simulink model "eVTOL_HIL"  (R2024b)
settings: Solver=FixedStepAuto  StartTime=0.0  StopTime=inf  FixedStep=SAMPLE_TIME  RelTol=1e-3
values from neighbouring files (symbols this model uses):
  aDl =     [initdata.mat]
  aDr =     [initdata.mat]
  aDyn =     [initdata.mat]
  aLat =     [initdata.mat]
  aLon =     [initdata.mat]
  D = Prop.D    [EOM_dt_MC.m]    (also in EOM_get_alf_dt_de_prop_evtol.m = CD * QS)
  General = init_layoutdata    [EOM_dt_MC.m]    (also in build_optimized_CA.m; initdata.mat = ; initdata_HIL_eVTOL.m)
  mass = Con(3)    [EOM_get_alf_dt_de_prop_evtol.m]    (also in initdata.mat = 2255.54; initdata_HIL_eVTOL.m = 7)
  Motor = init_motor_evtol    [EOM_dt_MC.m]    (also in initdata.mat = []; initdata_HIL_eVTOL.m)
  Prop = init_propeller_evtol_new    [EOM_dt_MC.m]    (also in initdata_HIL_eVTOL.m)
  SAMPLE_TIME = 0.01    [initdata_HIL_eVTOL.m]
undefined symbols (not defined in the file or in its folder): aDa, aDe, asbhl20env, Environment, InitData, magnitude
libraries: simulink_extras x16, vrlib x8, matrix_library x6, sharedutil x6, aerolibwindfilters x4, sharedtransform x4, aerolibfltsims x3, instrumentseriallib x3, uavmavlinklib x3, aerolibasang x3, aerolibobsolete x2, aerolibanimutils x1
(part 3 of 4)

== system eVTOL_HIL/eVTOL Dynamic Model/Energy & Power/thrust_6/Propeller  ==
  rpm : Inport
  V : Inport  Port=2
  rho : Inport  Port=3
  theta_b : Inport  Port=4
  D^5 : Constant  Value=5
  Diameter : Constant  Value=Prop.D
  Divide : Product  Inputs=4
  Divide2 : Product  Inputs=4
  Divide3 : Product  Inputs=**/
  Gain : Gain  Gain=1/60
  Math Function : Math  Operator=magnitude^2  SignedPower=on
  Math Function1 : Math  Operator=magnitude^2  SignedPower=on
  Math Function2 : Math  Operator=magnitude^2  SignedPower=on
  Math Function3 : Math  Operator=pow  SignedPower=on
  Math Function4 : Math  Operator=pow  SignedPower=on
  Scope{,1..4} (5 alike) : Scope
  Subsystem : Subsystem
  get CP : Lookup_n-D  BreakpointsForDimension1=Prop.J  BreakpointsForDimension2=Prop.theta_b  IndexSearchMethod=Linear search  BeginIndexSearchUsingPreviousIndexResult=on  Table=Prop.CP  RndMeth=Simplest
      settings: InputPortMap=u0,u1
  get CT : Lookup_n-D  BreakpointsForDimension1=Prop.J  BreakpointsForDimension2=Prop.theta_b  IndexSearchMethod=Linear search  BeginIndexSearchUsingPreviousIndexResult=on  Table=Prop.CT  RndMeth=Simplest
      settings: InputPortMap=u0,u1
  "n^3 " : Constant  Value=3
  P_plr (w) : Outport  VectorParamsAs1DForOutWhenUnconnected=off
  T (N) : Outport  Port=2  VectorParamsAs1DForOutWhenUnconnected=off
  eta_p : Outport  Port=3  VectorParamsAs1DForOutWhenUnconnected=off
  wires:
  Divide2/1 -> P_plr (w)/1, Scope/1
  Divide3/1 -> eta_p/1  "eta_p"
  D^5/1 -> Math Function4/2
  Math Function4/1 -> Divide2/4
  "n^3 "/1 -> Math Function3/2
  Math Function3/1 -> Divide2/3
  get CP/1 -> Divide3/3, Divide2/1, Scope3/1
  rpm/1 -> Gain/1, Subsystem/2(rpm)
  Subsystem/1(J) -> Scope2/1, get CT/1, Divide3/1, get CP/1
  Divide/1 -> Scope1/1, T (N)/1
  Math Function2/1 -> Divide/4  "D^4"
  Math Function1/1 -> Math Function2/1
  Diameter/1 -> Math Function1/1, Math Function4/1
  Math Function/1 -> Divide/3  "n^2"
  Gain/1 -> Math Function3/1, Math Function/1
  rho/1 -> Divide/2, Divide2/2
  get CT/1 -> Divide3/2, Divide/1, Scope4/1
  V/1 -> Subsystem/1(V)
  theta_b/1 -> get CP/2, get CT/2

== system eVTOL_HIL/eVTOL Dynamic Model/Environment/Wind Models/Dryden Wind Turbulence Model (Continuous (+q -r)) ==
  Altitude : Inport  Unit=m
  Airspeed : Inport  Port=2  Unit=m/s
  DCM : Inport  Port=3  Unit=1  PortDimensions=[3 3]
  (u,v,w) : Selector  InputPortWidth=4  IndexOptions=Index vector (dialog)  Indices=[1 2 3]  OutputSizes=1
  Angle Conversion : Subsystem
  Bus Creator : BusCreator  Inputs=3
  Cast : DataTypeConversion  SaturateOnIntegerOverflow=off  RndMeth=Floor
  Cast To Double{,1..4} (5 alike) : DataTypeConversion  OutDataTypeStr=double  SaturateOnIntegerOverflow=off  RndMeth=Floor
  Disallow CGS : UnitConfiguration  UnitSystemsStr=English,SI,SI (extended)  AllowAllUnitSystems=off
  Filters on angular rates : Subsystem  mask(Angular Rates){}
  Filters on velocities : aerolibwindfilters/Dryden Continuous Filters  SystemSampleTime=-1  VariantActivationTime=update diagram  AllowFlexibleInterface=on  Latency=0  AutoFrameSizeCalculation=off
  Length Conversion : Subsystem
  Length Conversion1 : Subsystem
  Mux : Mux  Inputs=3
  Mux1 : Mux  Inputs=3
  RMS turbulence intensities : Subsystem
  Select angular rates : Subsystem
  Select velocities : Subsystem
  Turbulence scale lengths : Subsystem
  Unit Conversion : UnitConversion  OutputType=Inherit: Inherit via back propagation
  Velocity Conversion : Subsystem
  Velocity Conversion2 : Subsystem
  White Noise : aerolibcommonsys/Tunable White Noise  pwr=[1 1 1 1]*pi  Ts=ts  seed=Seed
  Wind direction : Constant  Value=Wdeg
  Windspeed at 20ft (6m) : Constant  Value=W20
  Wingspan : Constant  Value=Wingspan
  p : Selector  InputPortWidth=4  IndexOptions=Index vector (dialog)  Indices=[4]  OutputSizes=1
  ug,vg,wg : Outport  Unit=m/s  VectorParamsAs1DForOutWhenUnconnected=off
  pg,qg,rg : Outport  Port=2  VectorParamsAs1DForOutWhenUnconnected=off
  wires:
  Cast To Double4/1 -> Velocity Conversion/1(in)
  Airspeed/1 -> Cast To Double4/1
  Cast To Double3/1 -> Length Conversion1/1(in)
  Wingspan/1 -> Cast To Double3/1
  Cast To Double2/1 -> Length Conversion/1(in)
  Cast To Double1/1 -> Angle Conversion/1(in)
  Cast To Double/1 -> Bus Creator/1  "DCM"
  Mux1/1 -> Cast/1
  Cast/1 -> pg,qg,rg/1
  (u,v,w)/1 -> Filters on velocities/1
  Unit Conversion/1 -> ug,vg,wg/1
  Velocity Conversion/1(out) -> Filters on angular rates/3(V), Filters on velocities/8
  Angle Conversion/1(out) -> Bus Creator/2  "Wdeg"
  Length Conversion1/1(out) -> Filters on angular rates/7(wingspan)
  Bus Creator/1 -> Select angular rates/4("DCM, altitude, Wdeg"), Select velocities/1("DCM, altitude, Wdeg")
  DCM/1 -> Cast To Double/1  "DCM"
  Wind direction/1 -> Cast To Double1/1
  Select angular rates/3(rgw) -> Mux1/3
  Select angular rates/2(qgw) -> Mux1/2
  Select angular rates/1(pgw) -> Mux1/1
  Select velocities/3(wgw) -> Mux/3
  Select velocities/2(vgw) -> Mux/2
  Select velocities/1(ugw) -> Mux/1
  Velocity Conversion2/1(out) -> RMS turbulence intensities/2(Windspeed at 20ft (6m))
  Windspeed at 20ft (6m)/1 -> Velocity Conversion2/1(in)
  RMS turbulence intensities/2(sigma_vg) -> Filters on velocities/6
  Filters on velocities/3 -> Filters on angular rates/2(wg), Select velocities/4(wgw_h&l)  "wgw"
  Filters on velocities/2 -> Filters on angular rates/1(vg), Select velocities/3(vgw_h&l)  "vgw"
  RMS turbulence intensities/1("sigma_ug ") -> Filters on velocities/5
  Filters on velocities/1 -> Select velocities/2(ugw_h&l)  "ugw"
  Filters on angular rates/3(rgw) -> Select angular rates/3(rgw_h&l)  "rgw"
  Filters on angular rates/2(qgw) -> Select angular rates/2(qgw_h&l)  "qgw"
  Filters on angular rates/1(pgw) -> Select angular rates/1(pgw_h&l)  "pgw"
  RMS turbulence intensities/3(sigma_wg) -> Filters on angular rates/5(sigma_w), Filters on velocities/7
  Turbulence scale lengths/3(L_wg) -> Filters on angular rates/4(Lw), Filters on velocities/4
  Turbulence scale lengths/1(L_ug) -> Filters on velocities/2
  Altitude/1 -> Cast To Double2/1
  Mux/1 -> Unit Conversion/1
  White Noise/1 -> (u,v,w)/1, p/1
  p/1 -> Filters on angular rates/6(Noise)
  Length Conversion/1(out) -> Bus Creator/3, RMS turbulence intensities/1(Altitude), Turbulence scale lengths/1(Altitude)  "altitude"
  Turbulence scale lengths/2(L_vg) -> Filters on velocities/3

== system eVTOL_HIL/eVTOL Dynamic Model/airframe/Flight Conditions/Subsystem2 ==
  Ve : Inport
  Dot Product1 : DotProduct  OutDataTypeStr=Inherit: Inherit via internal rule
  Gain1 : Gain  Gain=-1
  Selector4 : Selector  InputPortWidth=3  IndexOptions=Index vector (dialog)  Indices=3  OutputSizes=1
  Selector5 : Selector  InputPortWidth=3  IndexOptions=Index vector (dialog)  Indices=[1 2]  OutputSizes=1
  Selector6 : Selector  InputPortWidth=3  IndexOptions=Index vector (dialog)  Indices=2  OutputSizes=1
  Selector7 : Selector  InputPortWidth=3  IndexOptions=Index vector (dialog)  Indices=3  OutputSizes=1
  Sqrt1 : Sqrt
  Trigonometric Function2 : Trigonometry  Operator=atan2
  Trigonometric Function3 : Trigonometry  Operator=atan2
  gamma : Outport
  chi : Outport  Port=2
  wires:
  Ve/1 -> Selector7/1, Selector6/1, Selector5/1, Selector4/1
  Selector6/1 -> Trigonometric Function3/1
  Selector5/1 -> Dot Product1/1, Dot Product1/2
  Selector7/1 -> Trigonometric Function3/2
  Trigonometric Function2/1 -> gamma/1
  Gain1/1 -> Trigonometric Function2/1
  Dot Product1/1 -> Sqrt1/1
  Sqrt1/1 -> Trigonometric Function2/2
  Trigonometric Function3/1 -> chi/1
  Selector4/1 -> Gain1/1

== system eVTOL_HIL/eVTOL Dynamic Model/airframe/Flight Conditions/Vel in Inertial Axes ==
  Ve : Inport
  Demux : Demux  Outputs=3
  Dot Product1 : DotProduct  OutDataTypeStr=Inherit: Inherit via internal rule
  Fcn : Fcn  Expr=sqrt(u(1)^2+u(2)^2)
  Gain : Gain  Gain=3.6
  Mux : Mux  Inputs=2
  Mux1 : Mux  Inputs=5
  Sqrt : Sqrt
  Ve_Inertial : Outport  VectorParamsAs1DForOutWhenUnconnected=off
  wires:
  Demux/3 -> Mux1/3  "v_d"
  Ve/1 -> Demux/1, Dot Product1/2, Dot Product1/1
  Fcn/1 -> Mux1/4  "v_horizontal"
  Demux/1 -> Mux/1, Mux1/1  "v_n"
  Demux/2 -> Mux/2, Mux1/2  "v_e"
  Mux/1 -> Fcn/1
  Mux1/1 -> Ve_Inertial/1
  Gain/1 -> Mux1/5  "groundspeed(km/h)"
  Sqrt/1 -> Gain/1
  Dot Product1/1 -> Sqrt/1

== system eVTOL_HIL/eVTOL Dynamic Model/airframe/force moment/Gear&FM in body axis ==
  PlantData : Inport
  Add1 : Sum  Inputs=++++
  Add2 : Sum  Inputs=++++
  Constant1 : Constant  Value=0
  Constant6 : Constant  Value=0
  F 4 gear : Scope  NumInputPorts=4
  F&M  Front Gear Left : Subsystem
  F&M  Front Gear Right : Subsystem
  F&M  Main Gear Left : Subsystem
  F&M  Main Gear Right : Subsystem
  M 4 gear : Scope  NumInputPorts=4
  F_Gear : Outport  VectorParamsAs1DForOutWhenUnconnected=off
  M_Gear : Outport  Port=2  VectorParamsAs1DForOutWhenUnconnected=off
  wires:
  PlantData/1 -> F&M  Main Gear Right/1(PlantData), F&M  Main Gear Left/1(PlantData), F&M  Front Gear Right/1(PlantData), F&M  Front Gear Left/1(PlantData)
  F&M  Front Gear Left/2(M_fgl) -> M 4 gear/1, Add2/1
  F&M  Front Gear Left/1(F_fgl) -> F 4 gear/1, Add1/1
  F&M  Front Gear Right/1(F_fgl) -> F 4 gear/2, Add1/2
  F&M  Main Gear Left/1(F_fgl) -> F 4 gear/3, Add1/3
  F&M  Main Gear Right/1(F_fgl) -> F 4 gear/4, Add1/4
  Add1/1 -> F_Gear/1
  F&M  Front Gear Right/2(M_fgl) -> M 4 gear/2, Add2/2
  F&M  Main Gear Left/2(M_fgl) -> M 4 gear/3, Add2/3
  F&M  Main Gear Right/2(M_fgl) -> M 4 gear/4, Add2/4
  Add2/1 -> M_Gear/1
  Constant6/1 -> F&M  Main Gear Left/2(dg)
  Constant1/1 -> F&M  Main Gear Right/2(dg)

== system eVTOL_HIL/eVTOL Dynamic Model/airframe/force moment/Thrust&M in body axis ==
  prop : Inport
  3x3 Cross Product{,1..5} (6 alike) : sharedutil/3x3 Cross Product  aMode=aMode
  Bus Selector1 : BusSelector  OutputSignals=T_1,T_2,T_3,T_4,T_5,T_6,Q
  Constant1 : Constant  Value=General.pos_plr3
  Constant2 : Constant  Value=General.pos_plr4
  Constant3 : Constant  Value=General.pos_plr5
  Constant4 : Constant  Value=General.pos_plr1
  Constant5 : Constant  Value=General.pos_plr6
  Constant6 : Constant  Value=General.pos_plr2
  Display3 : Display
  Scope2 : Scope
  Sum2 : Sum  Inputs=++++++
  Sum3 : Sum  Inputs=++++++
  Sum4 : Sum  Inputs=++|
  T MC : Scope  NumInputPorts=6
  f_T : Outport  VectorParamsAs1DForOutWhenUnconnected=off
  m_T : Outport  Port=2  VectorParamsAs1DForOutWhenUnconnected=off
  wires:
  prop/1 -> Bus Selector1/1
  Constant4/1 -> 3x3 Cross Product/1
  Constant6/1 -> 3x3 Cross Product1/1
  Constant1/1 -> 3x3 Cross Product2/1
  Constant2/1 -> 3x3 Cross Product3/1
  Bus Selector1/1 -> T MC/1, [T_1]  "<T_1>"
  Bus Selector1/2 -> [T_2], T MC/2  "<T_2>"
  Bus Selector1/3 -> [T_3], T MC/3  "<T_3>"
  Bus Selector1/4 -> [T_4], T MC/4  "<T_4>"
  [T_1] -> 3x3 Cross Product/2
  [T_2] -> 3x3 Cross Product1/2
  [T_3] -> 3x3 Cross Product2/2
  [T_4] -> 3x3 Cross Product3/2
  [T_1] -> Sum2/1
  [T_2] -> Sum2/2
  [T_3] -> Sum2/3
  [T_4] -> Sum2/4
  3x3 Cross Product/1 -> Sum3/1
  3x3 Cross Product1/1 -> Sum3/2
  3x3 Cross Product2/1 -> Sum3/3
  3x3 Cross Product3/1 -> Sum3/4
  Sum2/1 -> f_T/1, Scope2/1, Display3/1  "T"
  Sum3/1 -> Sum4/2
  Bus Selector1/5 -> [T_5], T MC/5  "<T_5>"
  Sum4/1 -> m_T/1
  [Q] -> Sum4/1
  Bus Selector1/6 -> T MC/6, [T_6]  "<T_6>"
  Bus Selector1/7 -> [Q]  "<Q>"
  [T_5] -> Sum2/5
  [T_6] -> Sum2/6
  [T_5] -> 3x3 Cross Product4/2
  3x3 Cross Product4/1 -> Sum3/5
  Constant3/1 -> 3x3 Cross Product4/1
  [T_6] -> 3x3 Cross Product5/2
  3x3 Cross Product5/1 -> Sum3/6
  Constant5/1 -> 3x3 Cross Product5/1

== system eVTOL_HIL/eVTOL Dynamic Model/airframe/force moment/aero F&M in body axis ==
  PlantData : Inport
  Act_surface : Inport  Port=2
  Aerodynamic Coefficients : Subsystem  AncestorBlock=asbhl20vehicle/Vehicle/Aerodynamic/Aerodynamic Coefficients
      settings: LibrarySourceBlock=|
      | asbhl20vehicle/Vehicle/Aerodynamic/Aerodynamic
      | Coefficients
  "Aerodynamic Forces and Moments " : aerolibadyn/Aerodynamic Forces and Moments   inputAxes=Body  outputForceAxes=Body  outputMomentAxes=Body  S=General.Sw  b=General.b  cbar=General.MAC
  Center of Gravity : Constant  Value=[0 0 0]  SampleTime=0
  Center of Pressure : Constant  Value=[0 0 0]  SampleTime=0
  Constant : Constant
  Constant1 : Constant  Commented=on
  Mux1 : Mux  Inputs=2
  PlantBus : BusSelector  OutputSignals=Vb,alpha,beta,pqr,Va,alphaDot,mach
  PlantBus1 : BusSelector  OutputSignals=DynamicPressure
  PlantData_1 : InportShadow
  Product : Product
  Product1 : Product
  Scope1 : Scope  Commented=on
  Scope2 : Scope
  Scope3 : Scope
  Scope4 : Scope  Commented=on
  Selector : Selector  Commented=on  InputPortWidth=3  IndexOptions=Index vector (dialog)  Indices=1  OutputSizes=1
  Switch : Switch  Commented=on  Criteria=u2 > Threshold  Threshold=3  SaturateOnIntegerOverflow=off  InputSameDT=off
  nonunit value : Subsystem
  Fb (X Y Z) : Outport  VectorParamsAs1DForOutWhenUnconnected=off
  M (L M N) : Outport  Port=2  VectorParamsAs1DForOutWhenUnconnected=off
  wires:
  "Aerodynamic Forces and Moments "/1 -> Product/1, Scope2/1
  "Aerodynamic Forces and Moments "/2 -> Product1/1, Scope3/1
  PlantData/1 -> PlantBus/1
  Act_surface/1 -> Aerodynamic Coefficients/5(Act_surface)
  PlantBus/2 -> Mux1/1  "<alpha>"
  PlantBus/3 -> Mux1/2  "<beta>"
  PlantBus/4 -> nonunit value/2(pqr)  "<pqr>"
  Center of Gravity/1 -> "Aerodynamic Forces and Moments "/3
  Center of Pressure/1 -> "Aerodynamic Forces and Moments "/4
  PlantData_1/1 -> PlantBus1/1
  PlantBus/6 -> nonunit value/3(alphaDot)  "<alphaDot>"
  PlantBus/5 -> nonunit value/1(V)  "<Va>"
  Constant1/1 -> Switch/1
  Constant/1 -> [Aero_SW]
  Switch/1 -> Scope1/1
  Product/1 -> Fb (X Y Z)/1
  Product1/1 -> M (L M N)/1
  [Aero_SW] -> Product/2
  [Aero_SW] -> Product1/2
  PlantBus/1 -> Selector/1  "<Vb>"
  Selector/1 -> Switch/2, Scope4/1  "Vb_x"
  Mux1/1 -> Aerodynamic Coefficients/1(Incid)
  nonunit value/1(pqr_n) -> Aerodynamic Coefficients/3(pqrn)
  nonunit value/2(alphaDot_n) -> Aerodynamic Coefficients/4(alphaDot_n)
  Aerodynamic Coefficients/1(Coeff) -> "Aerodynamic Forces and Moments "/1
  PlantBus/7 -> Aerodynamic Coefficients/2(mach)  "<mach>"
  PlantBus1/1 -> "Aerodynamic Forces and Moments "/2  "<DynamicPressure>"

== system eVTOL_HIL/eVTOL Dynamic Model/airframe/force moment/gravity in body axis ==
  PlantData : Inport
  EnvmData : Inport  Port=2
  Bus Selector1 : BusSelector  OutputSignals=DCM_be,mass
  Bus Selector2 : BusSelector  OutputSignals=g
  G in body axis : Product  Multiplication=Matrix(*)  RndMeth=Zero
  Gain1 : Gain  Gain=[0; 0; 1]
  Product : Product  RndMeth=Zero
  Fb : Outport  VectorParamsAs1DForOutWhenUnconnected=off
  wires:
  Bus Selector1/1 -> G in body axis/1  "<DCM_be>"
  Gain1/1 -> G in body axis/2
  Bus Selector1/2 -> Product/1  "<mass>"
  Bus Selector2/1 -> Product/2  "<g>"
  Product/1 -> Gain1/1  "mg"
  PlantData/1 -> Bus Selector1/1
  G in body axis/1 -> Fb/1
  EnvmData/1 -> Bus Selector2/1

== system eVTOL_HIL/eVTOL Dynamic Model/Energy & Power/thrust_1/Propeller /Subsystem ==
  V : Inport
  rpm : Inport  Port=2
  Diameter : Constant  Value=Prop.D
  Divide : Product  Inputs=*//
  Gain : Gain  Gain=1/60
  J : Outport  VectorParamsAs1DForOutWhenUnconnected=off
  wires:
  Divide/1 -> J/1
  V/1 -> Divide/1
  rpm/1 -> Gain/1
  Gain/1 -> Divide/3  "rps"
  Diameter/1 -> Divide/2

== system eVTOL_HIL/eVTOL Dynamic Model/Energy & Power/thrust_2/Propeller /Subsystem ==
  V : Inport
  rpm : Inport  Port=2
  Diameter : Constant  Value=Prop.D
  Divide : Product  Inputs=*//
  Gain : Gain  Gain=1/60
  J : Outport  VectorParamsAs1DForOutWhenUnconnected=off
  wires:
  Divide/1 -> J/1
  V/1 -> Divide/1
  rpm/1 -> Gain/1
  Gain/1 -> Divide/3  "rps"
  Diameter/1 -> Divide/2

== system eVTOL_HIL/eVTOL Dynamic Model/Energy & Power/thrust_3/Propeller /Subsystem ==
  V : Inport
  rpm : Inport  Port=2
  Diameter : Constant  Value=Prop.D
  Divide : Product  Inputs=*//
  Gain : Gain  Gain=1/60
  J : Outport  VectorParamsAs1DForOutWhenUnconnected=off
  wires:
  Divide/1 -> J/1
  V/1 -> Divide/1
  rpm/1 -> Gain/1
  Gain/1 -> Divide/3  "rps"
  Diameter/1 -> Divide/2

== system eVTOL_HIL/eVTOL Dynamic Model/Energy & Power/thrust_4/Propeller /Subsystem ==
  V : Inport
  rpm : Inport  Port=2
  Diameter : Constant  Value=Prop.D
  Divide : Product  Inputs=*//
  Gain : Gain  Gain=1/60
  J : Outport  VectorParamsAs1DForOutWhenUnconnected=off
  wires:
  Divide/1 -> J/1
  V/1 -> Divide/1
  rpm/1 -> Gain/1
  Gain/1 -> Divide/3  "rps"
  Diameter/1 -> Divide/2

== system eVTOL_HIL/eVTOL Dynamic Model/Energy & Power/thrust_5/Propeller /Subsystem ==
  V : Inport
  rpm : Inport  Port=2
  Diameter : Constant  Value=Prop.D
  Divide : Product  Inputs=*//
  Gain : Gain  Gain=1/60
  J : Outport  VectorParamsAs1DForOutWhenUnconnected=off
  wires:
  Divide/1 -> J/1
  V/1 -> Divide/1
  rpm/1 -> Gain/1
  Gain/1 -> Divide/3  "rps"
  Diameter/1 -> Divide/2

== system eVTOL_HIL/eVTOL Dynamic Model/Energy & Power/thrust_6/Propeller /Subsystem ==
  V : Inport
  rpm : Inport  Port=2
  Diameter : Constant  Value=Prop.D
  Divide : Product  Inputs=*//
  Gain : Gain  Gain=1/60
  J : Outport  VectorParamsAs1DForOutWhenUnconnected=off
  wires:
  Divide/1 -> J/1
  V/1 -> Divide/1
  rpm/1 -> Gain/1
  Gain/1 -> Divide/3  "rps"
  Diameter/1 -> Divide/2

== system eVTOL_HIL/eVTOL Dynamic Model/Environment/Wind Models/Dryden Wind Turbulence Model (Continuous (+q -r))/Angle Conversion ==
  in : Inport  Unit=deg
  Unit Conversion : UnitConversion
  out : Outport  Unit=rad  VectorParamsAs1DForOutWhenUnconnected=off
  wires:
  in/1 -> Unit Conversion/1
  Unit Conversion/1 -> out/1

== system eVTOL_HIL/eVTOL Dynamic Model/Environment/Wind Models/Dryden Wind Turbulence Model (Continuous (+q -r))/Filters on angular rates ==
  vg : Inport
  wg : Inport  Port=2
  V : Inport  Port=3  Unit=ft/s
  Lw : Inport  Port=4
  sigma_w : Inport  Port=5
  Noise : Inport  Port=6
  wingspan : Inport  Port=7
  Constant1 : Constant  Value=T_on
  Constant2 : Constant  Value=T_on
  Constant3 : Constant  Value=T_on
  Hpgw : aerolibwindfilters/Hpgw(s)  SystemSampleTime=-1  VariantActivationTime=update diagram  AllowFlexibleInterface=on  Latency=0  AutoFrameSizeCalculation=off
  Hqgw : aerolibwindfilters/Hqgw(s) (+q)  SystemSampleTime=-1  VariantActivationTime=update diagram  AllowFlexibleInterface=on  Latency=0  AutoFrameSizeCalculation=off
  Hrgw : aerolibwindfilters/Hrgw(s) (-r)  SystemSampleTime=-1  VariantActivationTime=update diagram  AllowFlexibleInterface=on  Latency=0  AutoFrameSizeCalculation=off
  pgw : Outport  InitialOutput=0  VectorParamsAs1DForOutWhenUnconnected=off
  qgw : Outport  Port=2  InitialOutput=0  VectorParamsAs1DForOutWhenUnconnected=off
  rgw : Outport  Port=3  InitialOutput=0  VectorParamsAs1DForOutWhenUnconnected=off
  wires:
  Constant3/1 -> Hrgw/Enable
  Constant2/1 -> Hqgw/Enable
  Constant1/1 -> Hpgw/Enable
  Noise/1 -> Hpgw/3
  Lw/1 -> Hpgw/1
  sigma_w/1 -> Hpgw/2
  V/1 -> Hpgw/4, Hqgw/1, Hrgw/1
  Hpgw/1 -> pgw/1
  wg/1 -> Hqgw/2
  Hqgw/1 -> qgw/1
  Hrgw/1 -> rgw/1
  vg/1 -> Hrgw/2
  wingspan/1 -> Hqgw/3, Hrgw/3, Hpgw/5

== system eVTOL_HIL/eVTOL Dynamic Model/Environment/Wind Models/Dryden Wind Turbulence Model (Continuous (+q -r))/Length Conversion ==
  in : Inport
  Unit Conversion : UnitConversion
  out : Outport  Unit=ft  VectorParamsAs1DForOutWhenUnconnected=off
  wires:
  in/1 -> Unit Conversion/1
  Unit Conversion/1 -> out/1

== system eVTOL_HIL/eVTOL Dynamic Model/Environment/Wind Models/Dryden Wind Turbulence Model (Continuous (+q -r))/Length Conversion1 ==
  in : Inport  Unit=m
  Unit Conversion : UnitConversion
  out : Outport  Unit=ft  VectorParamsAs1DForOutWhenUnconnected=off
  wires:
  in/1 -> Unit Conversion/1
  Unit Conversion/1 -> out/1

== system eVTOL_HIL/eVTOL Dynamic Model/Environment/Wind Models/Dryden Wind Turbulence Model (Continuous (+q -r))/RMS turbulence intensities ==
  Altitude : Inport
  Windspeed at 20ft (6m) : Inport  Port=2
  High Altitude Intensity : Subsystem
  Low Altitude Intensity : Subsystem
  Mux1 : Mux  Inputs=2
  Mux2 : Mux  Inputs=2
  "sigma_ug " : Outport  VectorParamsAs1DForOutWhenUnconnected=off
  sigma_vg : Outport  Port=2  VectorParamsAs1DForOutWhenUnconnected=off
  sigma_wg : Outport  Port=3  VectorParamsAs1DForOutWhenUnconnected=off
  wires:
  Mux2/1 -> sigma_vg/1, "sigma_ug "/1  "sigmaug"
  Windspeed at 20ft (6m)/1 -> Low Altitude Intensity/1(Windspeed at 20ft (6m))
  High Altitude Intensity/1(sigma_ug sigma_vg sigma_wg) -> Mux2/2, Mux1/2
  Mux1/1 -> sigma_wg/1  "sigmawg"
  Low Altitude Intensity/2(sigma_wg) -> Mux1/1
  Low Altitude Intensity/1(sigma_ug sigma_vg) -> Mux2/1
  Altitude/1 -> High Altitude Intensity/1(h), Low Altitude Intensity/2(h)

== system eVTOL_HIL/eVTOL Dynamic Model/Environment/Wind Models/Dryden Wind Turbulence Model (Continuous (+q -r))/Select angular rates ==
  pgw_h&l : Inport
  qgw_h&l : Inport  Port=2
  rgw_h&l : Inport  Port=3
  "DCM, altitude, Wdeg" : Inport  Port=4
  Bus Creator : BusCreator  Inputs=6
  Bus Selector : BusSelector  OutputSignals=pgw,qgw,rgw
  Bus Selector1 : BusSelector  OutputSignals=pgw,qgw,rgw,DCM,Wdeg,altitude
  Bus Selector2 : BusSelector  OutputSignals=DCM,pgw,qgw,rgw,Wdeg
  Bus Selector3 : BusSelector  OutputSignals=altitude,DCM,Wdeg
  Interpolate rates : Subsystem  TreatAsAtomicUnit=on
  Low altitude rates : Subsystem  TreatAsAtomicUnit=on
  Medium/High altitude rates : Subsystem  TreatAsAtomicUnit=on
  Merge Subsystems : Subsystem
  "if Height < Max low altitude elseif Height > Min isotropic altitude " : If  IfExpression=u1<=max_height_low  ElseIfExpressions=u1>=min_height_high
  pgw : Outport  InitialOutput=0  VectorParamsAs1DForOutWhenUnconnected=off
  qgw : Outport  Port=2  InitialOutput=0  VectorParamsAs1DForOutWhenUnconnected=off
  rgw : Outport  Port=3  InitialOutput=0  VectorParamsAs1DForOutWhenUnconnected=off
  wires:
  "DCM, altitude, Wdeg"/1 -> Bus Selector3/1
  Bus Selector3/1 -> Bus Creator/1, "if Height < Max low altitude elseif Height > Min isotropic altitude "/1  "<altitude>"
  Bus Creator/1 -> Bus Selector2/1, Bus Selector1/1, Bus Selector/1
  Bus Selector3/2 -> Bus Creator/2  "<DCM>"
  pgw_h&l/1 -> Bus Creator/3
  qgw_h&l/1 -> Bus Creator/4
  rgw_h&l/1 -> Bus Creator/5
  Bus Selector1/1 -> Interpolate rates/1(pgw_h&l)  "<pgw>"
  Bus Selector1/2 -> Interpolate rates/2(qgw_h&l)  "<qgw>"
  Bus Selector1/3 -> Interpolate rates/3(rgw_h&l)  "<rgw>"
  Bus Selector1/4 -> Interpolate rates/4(DCM)  "<DCM>"
  Bus Selector1/6 -> Interpolate rates/6(Altitude)  "<altitude>"
  Bus Selector2/1 -> Low altitude rates/1(DCM)  "<DCM>"
  Bus Selector2/2 -> Low altitude rates/2(pgw_h&l)  "<pgw>"
  Bus Selector2/3 -> Low altitude rates/3(qgw_h&l)  "<qgw>"
  Bus Selector2/4 -> Low altitude rates/4(rgw_h&l)  "<rgw>"
  Bus Selector/1 -> Medium/High altitude rates/1(pgw_h&l)  "<pgw>"
  Bus Selector/2 -> Medium/High altitude rates/2(qgw_h&l)  "<qgw>"
  Bus Selector/3 -> Medium/High altitude rates/3(rgw_h&l)  "<rgw>"
  Merge Subsystems/1(pgw) -> pgw/1
  Merge Subsystems/2(qgw) -> qgw/1
  Merge Subsystems/3(rgw) -> rgw/1
  Interpolate rates/1(pgw,qgw,rgw) -> Merge Subsystems/3(interpolated)
  Bus Selector3/3 -> Bus Creator/6  "<Wdeg>"
  Bus Selector2/5 -> Low altitude rates/5(Wind direction)  "<Wdeg>"
  Bus Selector1/5 -> Interpolate rates/5(Wind direction)  "<Wdeg>"
  "if Height < Max low altitude elseif Height > Min isotropic altitude "/1 -> [IF]
  [IF] -> Low altitude rates/Action
  "if Height < Max low altitude elseif Height > Min isotropic altitude "/2 -> [ELSEIF]
  [ELSEIF] -> Medium/High altitude rates/Action
  [ELSE] -> Interpolate rates/Action
  "if Height < Max low altitude elseif Height > Min isotropic altitude "/3 -> [ELSE]
  Medium/High altitude rates/1(pgw,qgw,rgw) -> Merge Subsystems/2(high)
  Low altitude rates/1(pgw,qgw,rgw) -> Merge Subsystems/1(low)

== system eVTOL_HIL/eVTOL Dynamic Model/Environment/Wind Models/Dryden Wind Turbulence Model (Continuous (+q -r))/Select velocities ==
  "DCM, altitude, Wdeg" : Inport
  ugw_h&l : Inport  Port=2
  vgw_h&l : Inport  Port=3
  wgw_h&l : Inport  Port=4
  Bus Creator : BusCreator  Inputs=6
  Bus Selector : BusSelector  OutputSignals=ugw,vgw,wgw
  Bus Selector1 : BusSelector  OutputSignals=ugw,vgw,wgw,DCM,Wdeg,altitude
  Bus Selector2 : BusSelector  OutputSignals=DCM,ugw,vgw,wgw,Wdeg
  Bus Selector3 : BusSelector  OutputSignals=altitude,DCM,Wdeg
  Interpolate velocities : Subsystem  TreatAsAtomicUnit=on
  Low altitude velocities : Subsystem  TreatAsAtomicUnit=on
  Medium/High altitude velocities : Subsystem  TreatAsAtomicUnit=on
  Merge Subsystems : Subsystem
  "if Height < Max low altitude elseif Height > Min isotropic altitude " : If  IfExpression=u1<=max_height_low  ElseIfExpressions=u1>=min_height_high
  ugw : Outport  Unit=ft/s  InitialOutput=0  VectorParamsAs1DForOutWhenUnconnected=off
  vgw : Outport  Port=2  Unit=ft/s  InitialOutput=0  VectorParamsAs1DForOutWhenUnconnected=off
  wgw : Outport  Port=3  Unit=ft/s  InitialOutput=0  VectorParamsAs1DForOutWhenUnconnected=off
  wires:
  "DCM, altitude, Wdeg"/1 -> Bus Selector3/1
  Bus Selector1/6 -> Interpolate velocities/6(Altitude)  "<altitude>"
  Low altitude velocities/1(ugw,vgw,wgw) -> Merge Subsystems/1(low)
  Medium/High altitude velocities/1(ugw,vgw,wgw) -> Merge Subsystems/2(high)
  "if Height < Max low altitude elseif Height > Min isotropic altitude "/3 -> [ELSE]
  [ELSE] -> Interpolate velocities/Action
  [ELSEIF] -> Medium/High altitude velocities/Action
  "if Height < Max low altitude elseif Height > Min isotropic altitude "/2 -> [ELSEIF]
  [IF] -> Low altitude velocities/Action
  "if Height < Max low altitude elseif Height > Min isotropic altitude "/1 -> [IF]
  Bus Selector1/5 -> Interpolate velocities/5(Wind direction)  "<Wdeg>"
  Bus Selector2/5 -> Low altitude velocities/5(Wind direction)  "<Wdeg>"
  Bus Selector3/3 -> Bus Creator/6  "<Wdeg>"
  Interpolate velocities/1(ugw,vgw,wgw) -> Merge Subsystems/3(interpolated)
  Merge Subsystems/3(wgw) -> wgw/1
  Merge Subsystems/2(vgw) -> vgw/1
  Merge Subsystems/1(ugw) -> ugw/1
  Bus Selector/3 -> Medium/High altitude velocities/3(wgw_h&l)  "<wgw>"
  Bus Selector/2 -> Medium/High altitude velocities/2(vgw_h&l)  "<vgw>"
  Bus Selector/1 -> Medium/High altitude velocities/1(ugw_h&l)  "<ugw>"
  Bus Selector2/4 -> Low altitude velocities/4(wgw_h&l)  "<wgw>"
  Bus Selector2/3 -> Low altitude velocities/3(vgw_h&l)  "<vgw>"
  Bus Selector2/2 -> Low altitude velocities/2(ugw_h&l)  "<ugw>"
  Bus Selector2/1 -> Low altitude velocities/1(DCM)  "<DCM>"
  Bus Selector1/4 -> Interpolate velocities/4(DCM)  "<DCM>"
  Bus Selector1/3 -> Interpolate velocities/3(wgw_h&l)  "<wgw>"
  Bus Selector1/2 -> Interpolate velocities/2(vgw_h&l)  "<vgw>"
  Bus Selector1/1 -> Interpolate velocities/1(ugw_h&l)  "<ugw>"
  wgw_h&l/1 -> Bus Creator/5
  vgw_h&l/1 -> Bus Creator/4
  ugw_h&l/1 -> Bus Creator/3
  Bus Selector3/2 -> Bus Creator/2  "<DCM>"
  Bus Creator/1 -> Bus Selector2/1, Bus Selector/1, Bus Selector1/1
  Bus Selector3/1 -> Bus Creator/1, "if Height < Max low altitude elseif Height > Min isotropic altitude "/1  "<altitude>"

== system eVTOL_HIL/eVTOL Dynamic Model/Environment/Wind Models/Dryden Wind Turbulence Model (Continuous (+q -r))/Turbulence scale lengths ==
  Altitude : Inport
  Low altitude scale length : Subsystem
  Lv : Gain  SaturateOnIntegerOverflow=on  OutDataTypeStr=Inherit: Same as input  ParamDataTypeStr=Inherit: Same as input
  Lw : Gain  SaturateOnIntegerOverflow=on  OutDataTypeStr=Inherit: Same as input  ParamDataTypeStr=Inherit: Same as input
  Medium/High altitude scale length : Subsystem
  Mux : Mux  Inputs=2
  Mux1 : Mux  Inputs=2
  L_ug : Outport  VectorParamsAs1DForOutWhenUnconnected=off
  L_vg : Outport  Port=2  VectorParamsAs1DForOutWhenUnconnected=off
  L_wg : Outport  Port=3  VectorParamsAs1DForOutWhenUnconnected=off
  wires:
  Lv/1 -> L_vg/1
  Lw/1 -> L_wg/1
  Altitude/1 -> Low altitude scale length/1(h)
  Mux/1 -> Lw/1  "Lwg"
  Mux1/1 -> Lv/1, L_ug/1  "Lug"
  Low altitude scale length/1(L_ug L_vg) -> Mux1/1
  Low altitude scale length/2(L_wg) -> Mux/1
  Medium/High altitude scale length/1(L_ug L_vg L_wg) -> Mux1/2, Mux/2

== system eVTOL_HIL/eVTOL Dynamic Model/Environment/Wind Models/Dryden Wind Turbulence Model (Continuous (+q -r))/Velocity Conversion ==
  in : Inport
  Unit Conversion : UnitConversion
  out : Outport  Unit=ft/s  VectorParamsAs1DForOutWhenUnconnected=off
  wires:
  in/1 -> Unit Conversion/1
  Unit Conversion/1 -> out/1

== system eVTOL_HIL/eVTOL Dynamic Model/Environment/Wind Models/Dryden Wind Turbulence Model (Continuous (+q -r))/Velocity Conversion2 ==
  in : Inport  Unit=m/s
  Unit Conversion : UnitConversion
  out : Outport  Unit=ft/s  VectorParamsAs1DForOutWhenUnconnected=off
  wires:
  in/1 -> Unit Conversion/1
  Unit Conversion/1 -> out/1

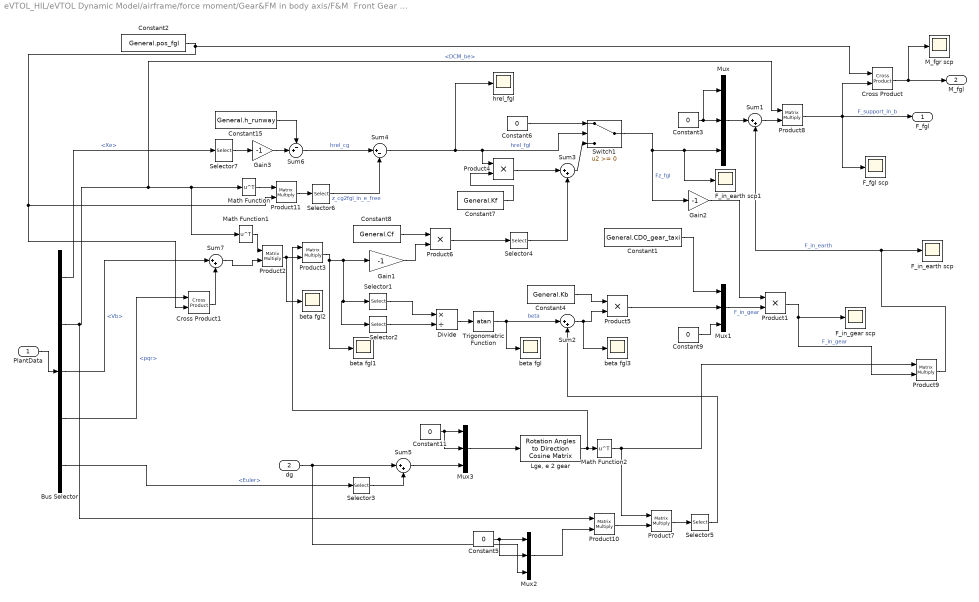
== system eVTOL_HIL/eVTOL Dynamic Model/airframe/force moment/Gear&FM in body axis/F&M  Front Gear Left ==
  PlantData : Inport
  dg : Inport  Port=2
  Bus Selector : BusSelector  OutputSignals=Xe,DCM_be,Vb,pqr,Euler
  Constant1 : Constant  Value=General.CD0_gear_taxi
  Constant{3,5..6,9,11} (5 alike) : Constant  Value=0
  Constant15 : Constant  Value=General.h_runway
  Constant2 : Constant  Value=General.pos_fgl
  Constant4 : Constant  Value=General.Kb
  Constant7 : Constant  Value=General.Kf
  Constant8 : Constant  Value=General.Cf
  Cross Product : vrlib/Utilities/Cross Product
  Cross Product1 : vrlib/Utilities/Cross Product
  Divide : Product  Inputs=*/
  F_fgl scp : Scope
  F_in_earth scp : Scope
  F_in_earth scp1 : Scope
  F_in_gear scp : Scope
  Gain1 : Gain  Gain=-1
  Gain2 : Gain  Gain=-1
  Gain3 : Gain  Gain=-1
  "Lge, e 2 gear" : sharedtransform/Rotation Angles to Direction Cosine Matrix  rotationOrder=XYZ  aMode=aMode
  M_fgr scp : Scope
  Math Function : Math  Operator=transpose  SignedPower=on
  Math Function1 : Math  Operator=transpose  SignedPower=on
  Math Function2 : Math  Operator=transpose  SignedPower=on
  Mux{,1..3} (4 alike) : Mux  Inputs=3
  Product{1,4..6} (4 alike) : Product
  Product{2..3,7..11} (7 alike) : Product  Multiplication=Matrix(*)
  Selector1 : Selector  InputPortWidth=3  IndexOptions=Index vector (dialog)  Indices=2  OutputSizes=1
  Selector2 : Selector  InputPortWidth=3  IndexOptions=Index vector (dialog)  Indices=1  OutputSizes=1
  Selector{3..7} (5 alike) : Selector  InputPortWidth=3  IndexOptions=Index vector (dialog)  Indices=3  OutputSizes=1
  Sum{1..3,5,7} (5 alike) : Sum  Inputs=|++
  Sum4 : Sum  Inputs=|+-
  Sum6 : Sum  Inputs=-+|
  Switch1 : Switch  SaturateOnIntegerOverflow=off  InputSameDT=off
  Trigonometric Function : Trigonometry  Operator=atan
  beta fgl{,1..3} (4 alike) : Scope
  hrel_fgl : Scope
  F_fgl : Outport  VectorParamsAs1DForOutWhenUnconnected=off
  M_fgl : Outport  Port=2  VectorParamsAs1DForOutWhenUnconnected=off
  wires:
  Selector5/1 -> Sum2/2
  Constant3/1 -> Mux/1, Mux/2
  Bus Selector/3 -> Sum7/1  "<Vb>"
  Product3/1 -> beta fgl1/1, Selector2/1, Selector1/1, Gain1/1
  Cross Product/1 -> M_fgl/1, M_fgr scp/1
  Math Function2/1 -> Product7/1, Product9/1
  Product5/1 -> Mux1/2
  dg/1 -> Mux2/3, Sum5/1
  Constant7/1 -> Product4/2
  Sum5/1 -> Mux3/3
  Constant5/1 -> Mux2/2, Mux2/1
  Sum1/1 -> Product8/2
  Constant4/1 -> Product5/1
  Selector4/1 -> Sum3/2
  Sum3/1 -> Switch1/3
  Constant11/1 -> Mux3/2, Mux3/1
  Mux/1 -> Sum1/1
  Mux3/1 -> "Lge, e 2 gear"/1
  Switch1/1 -> Gain2/1, F_in_earth scp1/1, Mux/3  "Fz_fgl"
  Constant1/1 -> Mux1/1
  Product6/1 -> Selector4/1
  Product10/1 -> Product7/2
  Selector3/1 -> Sum5/2
  "Lge, e 2 gear"/1 -> Product3/1, Math Function2/1
  Divide/1 -> Trigonometric Function/1
  Cross Product1/1 -> Sum7/2
  Constant6/1 -> Switch1/1
  Sum2/1 -> beta fgl3/1, Product5/2
  Product9/1 -> Sum1/2, F_in_earth scp/1  "F_in_earth"
  Product4/1 -> Sum3/1
  Selector1/1 -> Divide/1
  Product1/1 -> Product9/2, F_in_gear scp/1  "F_in_gear"
  Gain2/1 -> Product1/1
  Selector2/1 -> Divide/2
  Mux1/1 -> Product1/2  "F_in_gear"
  Gain1/1 -> Product6/2
  Constant9/1 -> Mux1/3
  Sum7/1 -> Product2/2
  Product8/1 -> F_fgl/1, F_fgl scp/1, Cross Product/2  "F_support_in_b"
  Mux2/1 -> Product10/2
  Bus Selector/5 -> Selector3/1  "<Euler>"
  Trigonometric Function/1 -> Sum2/1, beta fgl/1  "beta"
  Constant8/1 -> Product6/1
  Math Function1/1 -> Product2/1
  Product2/1 -> beta fgl2/1, Product3/2
  Bus Selector/4 -> Cross Product1/1  "<pqr>"
  Product7/1 -> Selector5/1
  Sum4/1 -> Product4/1, Switch1/2, hrel_fgl/1  "hrel_fgl"
  Bus Selector/1 -> Selector7/1  "<Xe>"
  Constant15/1 -> Sum6/1
  Selector6/1 -> Sum4/2  "z_cg2fgl_in_e_free"
  Product11/1 -> Selector6/1
  Selector7/1 -> Gain3/1
  Bus Selector/2 -> Product10/1, Product8/1, Math Function1/1, Math Function/1  "<DCM_be>"
  Math Function/1 -> Product11/1
  Gain3/1 -> Sum6/2
  Constant2/1 -> Cross Product/1, Product11/2, Cross Product1/2
  Sum6/1 -> Sum4/1  "hrel_cg"
  PlantData/1 -> Bus Selector/1

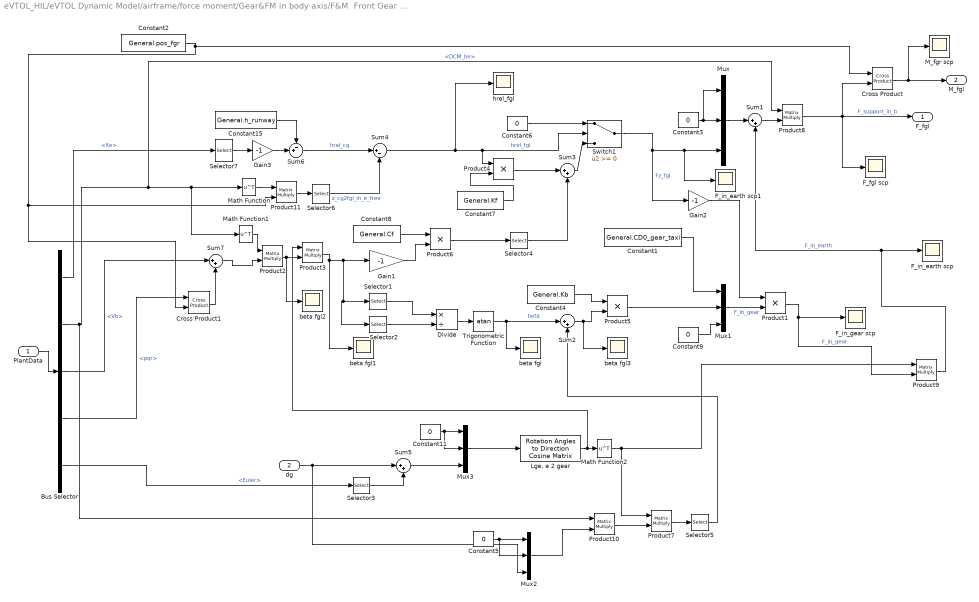
== system eVTOL_HIL/eVTOL Dynamic Model/airframe/force moment/Gear&FM in body axis/F&M  Front Gear Right ==
  PlantData : Inport
  dg : Inport  Port=2
  Bus Selector : BusSelector  OutputSignals=Xe,DCM_be,Vb,pqr,Euler
  Constant1 : Constant  Value=General.CD0_gear_taxi
  Constant{3,5..6,9,11} (5 alike) : Constant  Value=0
  Constant15 : Constant  Value=General.h_runway
  Constant2 : Constant  Value=General.pos_fgr
  Constant4 : Constant  Value=General.Kb
  Constant7 : Constant  Value=General.Kf
  Constant8 : Constant  Value=General.Cf
  Cross Product : vrlib/Utilities/Cross Product
  Cross Product1 : vrlib/Utilities/Cross Product
  Divide : Product  Inputs=*/
  F_fgl scp : Scope
  F_in_earth scp : Scope
  F_in_earth scp1 : Scope
  F_in_gear scp : Scope
  Gain1 : Gain  Gain=-1
  Gain2 : Gain  Gain=-1
  Gain3 : Gain  Gain=-1
  "Lge, e 2 gear" : sharedtransform/Rotation Angles to Direction Cosine Matrix  rotationOrder=XYZ  aMode=aMode
  M_fgr scp : Scope
  Math Function : Math  Operator=transpose  SignedPower=on
  Math Function1 : Math  Operator=transpose  SignedPower=on
  Math Function2 : Math  Operator=transpose  SignedPower=on
  Mux{,1..3} (4 alike) : Mux  Inputs=3
  Product{1,4..6} (4 alike) : Product
  Product{2..3,7..11} (7 alike) : Product  Multiplication=Matrix(*)
  Selector1 : Selector  InputPortWidth=3  IndexOptions=Index vector (dialog)  Indices=2  OutputSizes=1
  Selector2 : Selector  InputPortWidth=3  IndexOptions=Index vector (dialog)  Indices=1  OutputSizes=1
  Selector{3..7} (5 alike) : Selector  InputPortWidth=3  IndexOptions=Index vector (dialog)  Indices=3  OutputSizes=1
  Sum{1..3,5,7} (5 alike) : Sum  Inputs=|++
  Sum4 : Sum  Inputs=|+-
  Sum6 : Sum  Inputs=-+|
  Switch1 : Switch  SaturateOnIntegerOverflow=off  InputSameDT=off
  Trigonometric Function : Trigonometry  Operator=atan
  beta fgl{,1..3} (4 alike) : Scope
  hrel_fgl : Scope
  F_fgl : Outport  VectorParamsAs1DForOutWhenUnconnected=off
  M_fgl : Outport  Port=2  VectorParamsAs1DForOutWhenUnconnected=off
  wires:
  Selector5/1 -> Sum2/2
  Constant3/1 -> Mux/1, Mux/2
  Bus Selector/3 -> Sum7/1  "<Vb>"
  Product3/1 -> beta fgl1/1, Selector2/1, Selector1/1, Gain1/1
  Cross Product/1 -> M_fgl/1, M_fgr scp/1
  Math Function2/1 -> Product7/1, Product9/1
  Product5/1 -> Mux1/2
  dg/1 -> Mux2/3, Sum5/1
  Constant7/1 -> Product4/2
  Sum5/1 -> Mux3/3
  Constant5/1 -> Mux2/2, Mux2/1
  Sum1/1 -> Product8/2
  Constant4/1 -> Product5/1
  Selector4/1 -> Sum3/2
  Sum3/1 -> Switch1/3
  Constant11/1 -> Mux3/2, Mux3/1
  Mux/1 -> Sum1/1
  Mux3/1 -> "Lge, e 2 gear"/1
  Switch1/1 -> Gain2/1, F_in_earth scp1/1, Mux/3  "Fz_fgl"
  Constant1/1 -> Mux1/1
  Product6/1 -> Selector4/1
  Product10/1 -> Product7/2
  Selector3/1 -> Sum5/2
  "Lge, e 2 gear"/1 -> Product3/1, Math Function2/1
  Divide/1 -> Trigonometric Function/1
  Cross Product1/1 -> Sum7/2
  Constant6/1 -> Switch1/1
  Sum2/1 -> beta fgl3/1, Product5/2
  Product9/1 -> Sum1/2, F_in_earth scp/1  "F_in_earth"
  Product4/1 -> Sum3/1
  Selector1/1 -> Divide/1
  Product1/1 -> Product9/2, F_in_gear scp/1  "F_in_gear"
  Gain2/1 -> Product1/1
  Selector2/1 -> Divide/2
  Mux1/1 -> Product1/2  "F_in_gear"
  Gain1/1 -> Product6/2
  Constant9/1 -> Mux1/3
  Sum7/1 -> Product2/2
  Product8/1 -> F_fgl/1, F_fgl scp/1, Cross Product/2  "F_support_in_b"
  Mux2/1 -> Product10/2
  Bus Selector/5 -> Selector3/1  "<Euler>"
  Trigonometric Function/1 -> Sum2/1, beta fgl/1  "beta"
  Constant8/1 -> Product6/1
  Math Function1/1 -> Product2/1
  Product2/1 -> beta fgl2/1, Product3/2
  Bus Selector/4 -> Cross Product1/1  "<pqr>"
  Product7/1 -> Selector5/1
  Sum4/1 -> Product4/1, Switch1/2, hrel_fgl/1  "hrel_fgl"
  Bus Selector/1 -> Selector7/1  "<Xe>"
  Constant15/1 -> Sum6/1
  Selector6/1 -> Sum4/2  "z_cg2fgl_in_e_free"
  Product11/1 -> Selector6/1
  Selector7/1 -> Gain3/1
  Bus Selector/2 -> Product10/1, Product8/1, Math Function1/1, Math Function/1  "<DCM_be>"
  Math Function/1 -> Product11/1
  Gain3/1 -> Sum6/2
  Constant2/1 -> Cross Product/1, Product11/2, Cross Product1/2
  Sum6/1 -> Sum4/1  "hrel_cg"
  PlantData/1 -> Bus Selector/1

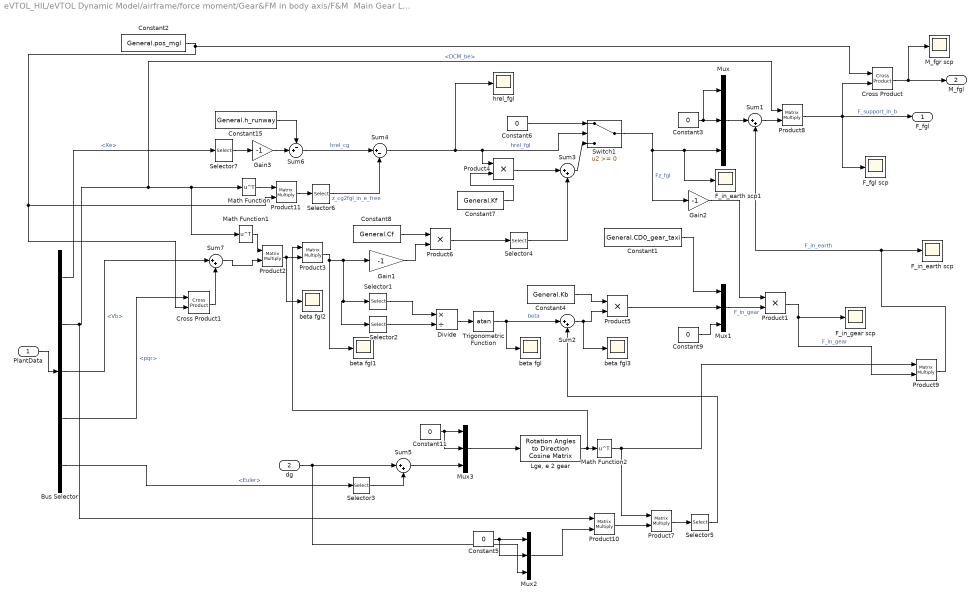
== system eVTOL_HIL/eVTOL Dynamic Model/airframe/force moment/Gear&FM in body axis/F&M  Main Gear Left ==
  PlantData : Inport
  dg : Inport  Port=2
  Bus Selector : BusSelector  OutputSignals=Xe,DCM_be,Vb,pqr,Euler
  Constant1 : Constant  Value=General.CD0_gear_taxi
  Constant{3,5..6,9,11} (5 alike) : Constant  Value=0
  Constant15 : Constant  Value=General.h_runway
  Constant2 : Constant  Value=General.pos_mgl
  Constant4 : Constant  Value=General.Kb
  Constant7 : Constant  Value=General.Kf
  Constant8 : Constant  Value=General.Cf
  Cross Product : vrlib/Utilities/Cross Product
  Cross Product1 : vrlib/Utilities/Cross Product
  Divide : Product  Inputs=*/
  F_fgl scp : Scope
  F_in_earth scp : Scope
  F_in_earth scp1 : Scope
  F_in_gear scp : Scope
  Gain1 : Gain  Gain=-1
  Gain2 : Gain  Gain=-1
  Gain3 : Gain  Gain=-1
  "Lge, e 2 gear" : sharedtransform/Rotation Angles to Direction Cosine Matrix  rotationOrder=XYZ  aMode=aMode
  M_fgr scp : Scope
  Math Function : Math  Operator=transpose  SignedPower=on
  Math Function1 : Math  Operator=transpose  SignedPower=on
  Math Function2 : Math  Operator=transpose  SignedPower=on
  Mux{,1..3} (4 alike) : Mux  Inputs=3
  Product{1,4..6} (4 alike) : Product
  Product{2..3,7..11} (7 alike) : Product  Multiplication=Matrix(*)
  Selector1 : Selector  InputPortWidth=3  IndexOptions=Index vector (dialog)  Indices=2  OutputSizes=1
  Selector2 : Selector  InputPortWidth=3  IndexOptions=Index vector (dialog)  Indices=1  OutputSizes=1
  Selector{3..7} (5 alike) : Selector  InputPortWidth=3  IndexOptions=Index vector (dialog)  Indices=3  OutputSizes=1
  Sum{1..3,5,7} (5 alike) : Sum  Inputs=|++
  Sum4 : Sum  Inputs=|+-
  Sum6 : Sum  Inputs=-+|
  Switch1 : Switch  SaturateOnIntegerOverflow=off  InputSameDT=off
  Trigonometric Function : Trigonometry  Operator=atan
  beta fgl{,1..3} (4 alike) : Scope
  hrel_fgl : Scope
  F_fgl : Outport  VectorParamsAs1DForOutWhenUnconnected=off
  M_fgl : Outport  Port=2  VectorParamsAs1DForOutWhenUnconnected=off
  wires:
  Selector5/1 -> Sum2/2
  Constant3/1 -> Mux/1, Mux/2
  Bus Selector/3 -> Sum7/1  "<Vb>"
  Product3/1 -> beta fgl1/1, Selector2/1, Selector1/1, Gain1/1
  Cross Product/1 -> M_fgl/1, M_fgr scp/1
  Math Function2/1 -> Product7/1, Product9/1
  Product5/1 -> Mux1/2
  dg/1 -> Mux2/3, Sum5/1
  Constant7/1 -> Product4/2
  Sum5/1 -> Mux3/3
  Constant5/1 -> Mux2/2, Mux2/1
  Sum1/1 -> Product8/2
  Constant4/1 -> Product5/1
  Selector4/1 -> Sum3/2
  Sum3/1 -> Switch1/3
  Constant11/1 -> Mux3/2, Mux3/1
  Mux/1 -> Sum1/1
  Mux3/1 -> "Lge, e 2 gear"/1
  Switch1/1 -> Gain2/1, F_in_earth scp1/1, Mux/3  "Fz_fgl"
  Constant1/1 -> Mux1/1
  Product6/1 -> Selector4/1
  Product10/1 -> Product7/2
  Selector3/1 -> Sum5/2
  "Lge, e 2 gear"/1 -> Product3/1, Math Function2/1
  Divide/1 -> Trigonometric Function/1
  Cross Product1/1 -> Sum7/2
  Constant6/1 -> Switch1/1
  Sum2/1 -> beta fgl3/1, Product5/2
  Product9/1 -> Sum1/2, F_in_earth scp/1  "F_in_earth"
  Product4/1 -> Sum3/1
  Selector1/1 -> Divide/1
  Product1/1 -> Product9/2, F_in_gear scp/1  "F_in_gear"
  Gain2/1 -> Product1/1
  Selector2/1 -> Divide/2
  Mux1/1 -> Product1/2  "F_in_gear"
  Gain1/1 -> Product6/2
  Constant9/1 -> Mux1/3
  Sum7/1 -> Product2/2
  Product8/1 -> F_fgl/1, F_fgl scp/1, Cross Product/2  "F_support_in_b"
  Mux2/1 -> Product10/2
  Bus Selector/5 -> Selector3/1  "<Euler>"
  Trigonometric Function/1 -> Sum2/1, beta fgl/1  "beta"
  Constant8/1 -> Product6/1
  Math Function1/1 -> Product2/1
  Product2/1 -> beta fgl2/1, Product3/2
  Bus Selector/4 -> Cross Product1/1  "<pqr>"
  Product7/1 -> Selector5/1
  Sum4/1 -> Product4/1, Switch1/2, hrel_fgl/1  "hrel_fgl"
  Bus Selector/1 -> Selector7/1  "<Xe>"
  Constant15/1 -> Sum6/1
  Selector6/1 -> Sum4/2  "z_cg2fgl_in_e_free"
  Product11/1 -> Selector6/1
  Selector7/1 -> Gain3/1
  Bus Selector/2 -> Product10/1, Product8/1, Math Function1/1, Math Function/1  "<DCM_be>"
  Math Function/1 -> Product11/1
  Gain3/1 -> Sum6/2
  Constant2/1 -> Cross Product/1, Product11/2, Cross Product1/2
  Sum6/1 -> Sum4/1  "hrel_cg"
  PlantData/1 -> Bus Selector/1

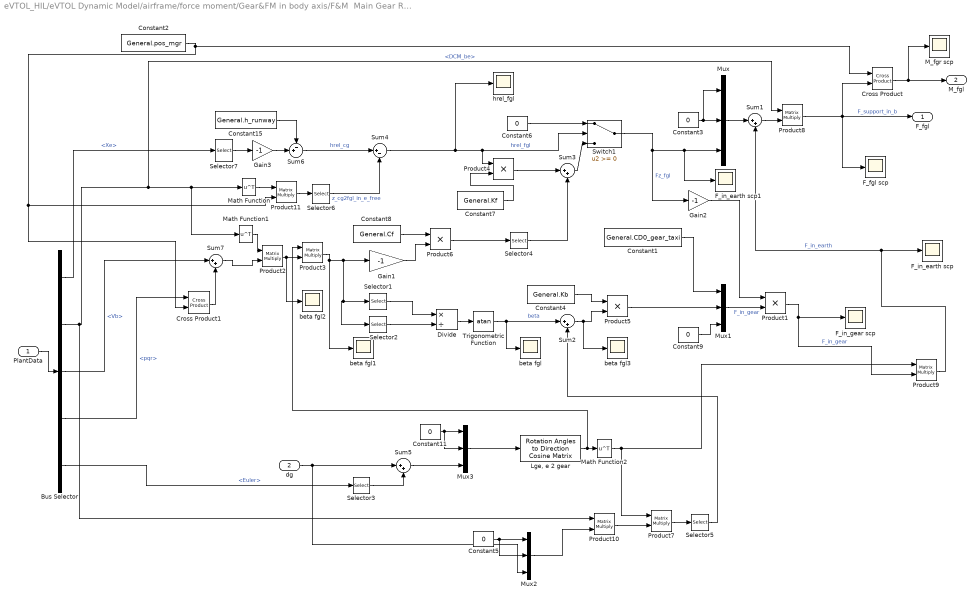
== system eVTOL_HIL/eVTOL Dynamic Model/airframe/force moment/Gear&FM in body axis/F&M  Main Gear Right ==
  PlantData : Inport
  dg : Inport  Port=2
  Bus Selector : BusSelector  OutputSignals=Xe,DCM_be,Vb,pqr,Euler
  Constant1 : Constant  Value=General.CD0_gear_taxi
  Constant{3,5..6,9,11} (5 alike) : Constant  Value=0
  Constant15 : Constant  Value=General.h_runway
  Constant2 : Constant  Value=General.pos_mgr
  Constant4 : Constant  Value=General.Kb
  Constant7 : Constant  Value=General.Kf
  Constant8 : Constant  Value=General.Cf
  Cross Product : vrlib/Utilities/Cross Product
  Cross Product1 : vrlib/Utilities/Cross Product
  Divide : Product  Inputs=*/
  F_fgl scp : Scope
  F_in_earth scp : Scope
  F_in_earth scp1 : Scope
  F_in_gear scp : Scope
  Gain1 : Gain  Gain=-1
  Gain2 : Gain  Gain=-1
  Gain3 : Gain  Gain=-1
  "Lge, e 2 gear" : sharedtransform/Rotation Angles to Direction Cosine Matrix  rotationOrder=XYZ  aMode=aMode
  M_fgr scp : Scope
  Math Function : Math  Operator=transpose  SignedPower=on
  Math Function1 : Math  Operator=transpose  SignedPower=on
  Math Function2 : Math  Operator=transpose  SignedPower=on
  Mux{,1..3} (4 alike) : Mux  Inputs=3
  Product{1,4..6} (4 alike) : Product
  Product{2..3,7..11} (7 alike) : Product  Multiplication=Matrix(*)
  Selector1 : Selector  InputPortWidth=3  IndexOptions=Index vector (dialog)  Indices=2  OutputSizes=1
  Selector2 : Selector  InputPortWidth=3  IndexOptions=Index vector (dialog)  Indices=1  OutputSizes=1
  Selector{3..7} (5 alike) : Selector  InputPortWidth=3  IndexOptions=Index vector (dialog)  Indices=3  OutputSizes=1
  Sum{1..3,5,7} (5 alike) : Sum  Inputs=|++
  Sum4 : Sum  Inputs=|+-
  Sum6 : Sum  Inputs=-+|
  Switch1 : Switch  SaturateOnIntegerOverflow=off  InputSameDT=off
  Trigonometric Function : Trigonometry  Operator=atan
  beta fgl{,1..3} (4 alike) : Scope
  hrel_fgl : Scope
  F_fgl : Outport  VectorParamsAs1DForOutWhenUnconnected=off
  M_fgl : Outport  Port=2  VectorParamsAs1DForOutWhenUnconnected=off
  wires:
  Selector5/1 -> Sum2/2
  Constant3/1 -> Mux/1, Mux/2
  Bus Selector/3 -> Sum7/1  "<Vb>"
  Product3/1 -> beta fgl1/1, Selector2/1, Selector1/1, Gain1/1
  Cross Product/1 -> M_fgl/1, M_fgr scp/1
  Math Function2/1 -> Product7/1, Product9/1
  Product5/1 -> Mux1/2
  dg/1 -> Mux2/3, Sum5/1
  Constant7/1 -> Product4/2
  Sum5/1 -> Mux3/3
  Constant5/1 -> Mux2/2, Mux2/1
  Sum1/1 -> Product8/2
  Constant4/1 -> Product5/1
  Selector4/1 -> Sum3/2
  Sum3/1 -> Switch1/3
  Constant11/1 -> Mux3/2, Mux3/1
  Mux/1 -> Sum1/1
  Mux3/1 -> "Lge, e 2 gear"/1
  Switch1/1 -> Gain2/1, F_in_earth scp1/1, Mux/3  "Fz_fgl"
  Constant1/1 -> Mux1/1
  Product6/1 -> Selector4/1
  Product10/1 -> Product7/2
  Selector3/1 -> Sum5/2
  "Lge, e 2 gear"/1 -> Product3/1, Math Function2/1
  Divide/1 -> Trigonometric Function/1
  Cross Product1/1 -> Sum7/2
  Constant6/1 -> Switch1/1
  Sum2/1 -> beta fgl3/1, Product5/2
  Product9/1 -> Sum1/2, F_in_earth scp/1  "F_in_earth"
  Product4/1 -> Sum3/1
  Selector1/1 -> Divide/1
  Product1/1 -> Product9/2, F_in_gear scp/1  "F_in_gear"
  Gain2/1 -> Product1/1
  Selector2/1 -> Divide/2
  Mux1/1 -> Product1/2  "F_in_gear"
  Gain1/1 -> Product6/2
  Constant9/1 -> Mux1/3
  Sum7/1 -> Product2/2
  Product8/1 -> F_fgl/1, F_fgl scp/1, Cross Product/2  "F_support_in_b"
  Mux2/1 -> Product10/2
  Bus Selector/5 -> Selector3/1  "<Euler>"
  Trigonometric Function/1 -> Sum2/1, beta fgl/1  "beta"
  Constant8/1 -> Product6/1
  Math Function1/1 -> Product2/1
  Product2/1 -> beta fgl2/1, Product3/2
  Bus Selector/4 -> Cross Product1/1  "<pqr>"
  Product7/1 -> Selector5/1
  Sum4/1 -> Product4/1, Switch1/2, hrel_fgl/1  "hrel_fgl"
  Bus Selector/1 -> Selector7/1  "<Xe>"
  Constant15/1 -> Sum6/1
  Selector6/1 -> Sum4/2  "z_cg2fgl_in_e_free"
  Product11/1 -> Selector6/1
  Selector7/1 -> Gain3/1
  Bus Selector/2 -> Product10/1, Product8/1, Math Function1/1, Math Function/1  "<DCM_be>"
  Math Function/1 -> Product11/1
  Gain3/1 -> Sum6/2
  Constant2/1 -> Cross Product/1, Product11/2, Cross Product1/2
  Sum6/1 -> Sum4/1  "hrel_cg"
  PlantData/1 -> Bus Selector/1

== system eVTOL_HIL/eVTOL Dynamic Model/airframe/force moment/aero F&M in body axis/Aerodynamic Coefficients ==
  Incid : Inport
  mach : Inport  Port=2
  pqrn : Inport  Port=3
  alphaDot_n : Inport  Port=4
  Act_surface : Inport  Port=5
  Actuator Increments : Subsystem  AncestorBlock=|
      | asbhl20vehicle/Vehicle/Aerodynamic/Aerodynamic
      | Coefficients/Actuator
      | Increments
      settings: LibrarySourceBlock=|
      | asbhl20vehicle/Vehicle/Aerodynamic/Aerodynamic
      | Coefficients/Actuator
      | Increments
  Basic Coefficients : Subsystem  AncestorBlock=asbhl20vehicle/Vehicle/Aerodynamic/Aerodynamic Coefficients/Datum Coefficients
      settings: LibrarySourceBlock=|
      | asbhl20vehicle/Vehicle/Aerodynamic/Aerodynamic
      | Coefficients/Datum Coefficients
  Body Rate Damping : Subsystem  AncestorBlock=|
      | asbhl20vehicle/Vehicle/Aerodynamic/Aerodynamic
      | Coefficients/Body Rate
      | Damping
      settings: LibrarySourceBlock=|
      | asbhl20vehicle/Vehicle/Aerodynamic/Aerodynamic
      | Coefficients/Body Rate
      | Damping
  CLCDCY-CXCYCZ : Subsystem
  Divide : Product  Inputs=*/
  K : Scope
  Mux1 : Mux  Inputs=2
  Scope{1..5} (5 alike) : Scope
  Selector : Selector  InputPortWidth=6  IndexOptions=Index vector (dialog)  Indices=[1 2 3]  OutputSizes=1
  Selector1 : Selector  InputPortWidth=6  IndexOptions=Index vector (dialog)  Indices=[4 5 6]  OutputSizes=1
  Selector2 : Selector  InputPortWidth=3  IndexOptions=Index vector (dialog)  Indices=1  OutputSizes=1
  Selector3 : Selector  InputPortWidth=3  IndexOptions=Index vector (dialog)  Indices=2  OutputSizes=1
  Sum : Sum  Inputs=3  InputSameDT=on  SaturateOnIntegerOverflow=on  OutDataTypeStr=Inherit: Same as first input
  Coeff : Outport  InitialOutput=0  VectorParamsAs1DForOutWhenUnconnected=off
  wires:
  CLCDCY-CXCYCZ/1(Cl_XYZ) -> Scope1/1, Mux1/1
  Selector1/1 -> Mux1/2, Scope5/1
  Basic Coefficients/1(cl) -> Sum/1, Scope2/1
  Selector2/1 -> Divide/1  "CL"
  Body Rate Damping/1(cl) -> Sum/3, Scope4/1
  alphaDot_n/1 -> Body Rate Damping/3(alphaDot_n)
  Mux1/1 -> Coeff/1
  pqrn/1 -> Body Rate Damping/2(pqrn)
  Actuator Increments/1(cl) -> Sum/2, Scope3/1
  Selector/1 -> Selector3/1, Selector2/1, CLCDCY-CXCYCZ/2(Cl_LDY)
  Selector3/1 -> Divide/2  "CD"
  Sum/1 -> Selector/1, Selector1/1
  Divide/1 -> K/1
  Incid/1 -> Actuator Increments/2(incid), CLCDCY-CXCYCZ/1(Incid), Body Rate Damping/1(Incid), Basic Coefficients/1(Incid)
  Act_surface/1 -> Actuator Increments/1(Actuators)
  mach/1 -> Basic Coefficients/2(mach)
